simulink model "freq_exec"  (Simulink 3.00)
libraries: execlib x5

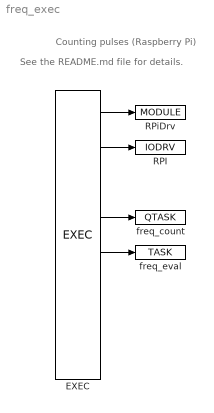
== system freq_exec ==
  note: See the README.md file for details.
  note: Counting pulses (Raspberry Pi)
  EXEC : execlib/EXEC  target=Generic target device  tick=0.002  ntick0=50  ntick1=50  ntick2=100  ntick3=1200  pri0=5  pri1=9  pri2=13  pri3=18
  RPI : execlib/IODRV  module=RPiDrv  classname=RPiDrv  factor=1  stack=10240  pri=3  timer=off
  RPiDrv : execlib/MODULE
  freq_count : execlib/QTASK  factor=1  stack=10240  MDLOPEN=on
  freq_eval : execlib/TASK  factor=1  start=0  stop=1  stack=10240  MDLOPEN=on
  wires:
  EXEC/1 -> RPiDrv/1
  EXEC/2 -> RPI/1
  EXEC/4 -> freq_count/1
  EXEC/5 -> freq_eval/1
